simulink model "AEKF_Digital_Twin"  (R2026a)
settings: Solver=ode1  StopTime=T_sim  FixedStep=0.002
settings Model: Creator=Adham  LastModifiedBy=Adham

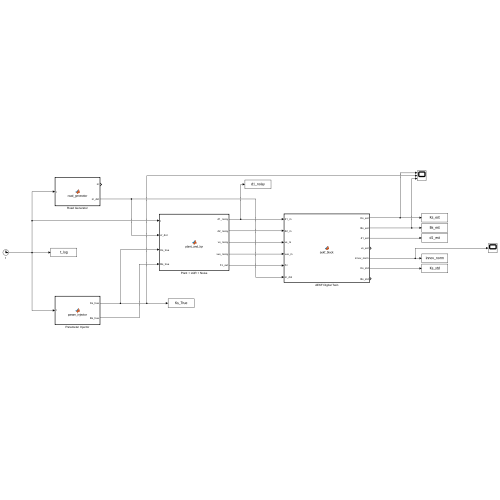
[thumbnail: Simulink's stored preview of the top-level diagram]
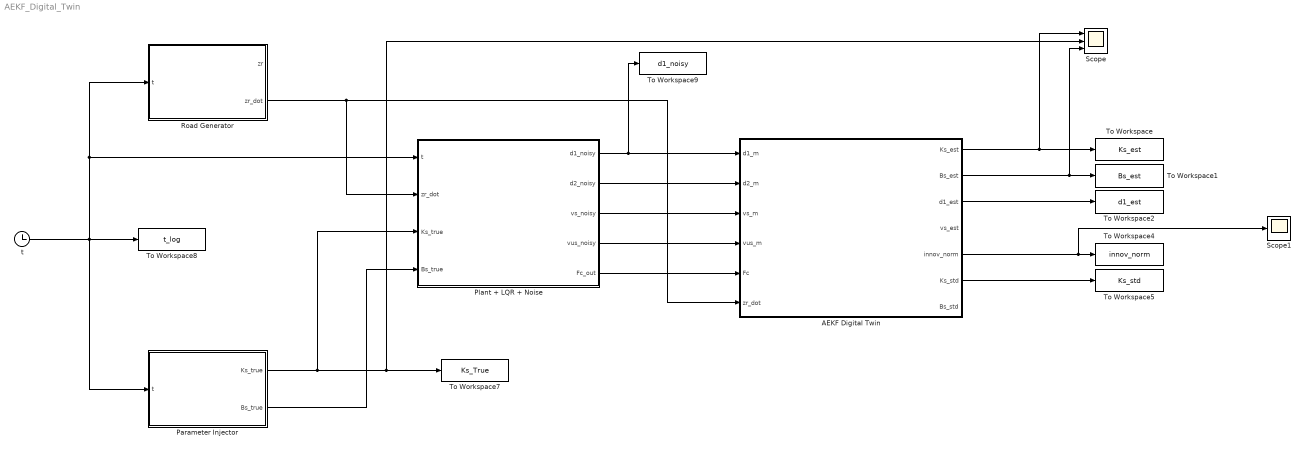
== system AEKF_Digital_Twin ==
  AEKF Digital Twin : MATLAB Function  TreatAsAtomicUnit=on
  Parameter Injector : MATLAB Function  TreatAsAtomicUnit=on
  Plant + LQR + Noise : MATLAB Function  TreatAsAtomicUnit=on
  Road Generator : MATLAB Function  TreatAsAtomicUnit=on
  Scope : Scope  NumInputPorts=3
  Scope1 : Scope
  To Workspace : ToWorkspace  VariableName=Ks_est  SaveFormat=Timeseries  SampleTime=-1
  To Workspace1 : ToWorkspace  VariableName=Bs_est  SaveFormat=Timeseries  SampleTime=-1
  To Workspace2 : ToWorkspace  VariableName=d1_est  SaveFormat=Timeseries  SampleTime=-1
  To Workspace4 : ToWorkspace  VariableName=innov_norm  SaveFormat=Timeseries  SampleTime=-1
  To Workspace5 : ToWorkspace  VariableName=Ks_std  SaveFormat=Timeseries  SampleTime=-1
  To Workspace7 : ToWorkspace  VariableName=Ks_True  SaveFormat=Timeseries  SampleTime=-1
  To Workspace8 : ToWorkspace  VariableName=t_log  SaveFormat=Timeseries  SampleTime=-1
  To Workspace9 : ToWorkspace  VariableName=d1_noisy  SaveFormat=Timeseries  SampleTime=-1
  t : Clock
  wires:
  t/1 -> To Workspace8/1, Road Generator/1(t), Plant + LQR + Noise/1(t), Parameter Injector/1(t)
  Parameter Injector/1(Ks_true) -> To Workspace7/1, Scope/2, Plant + LQR + Noise/3(Ks_true)
  Parameter Injector/2(Bs_true) -> Plant + LQR + Noise/4(Bs_true)
  Plant + LQR + Noise/1(d1_noisy) -> To Workspace9/1, AEKF Digital Twin/1(d1_m)
  Plant + LQR + Noise/2(d2_noisy) -> AEKF Digital Twin/2(d2_m)
  Plant + LQR + Noise/3(vs_noisy) -> AEKF Digital Twin/3(vs_m)
  Plant + LQR + Noise/4(vus_noisy) -> AEKF Digital Twin/4(vus_m)
  Plant + LQR + Noise/5(Fc_out) -> AEKF Digital Twin/5(Fc)
  Road Generator/2(zr_dot) -> AEKF Digital Twin/6(zr_dot), Plant + LQR + Noise/2(zr_dot)
  AEKF Digital Twin/1(Ks_est) -> Scope/1, To Workspace/1
  AEKF Digital Twin/2(Bs_est) -> Scope/3, To Workspace1/1
  AEKF Digital Twin/5(innov_norm) -> Scope1/1, To Workspace4/1
  AEKF Digital Twin/6(Ks_std) -> To Workspace5/1
  AEKF Digital Twin/3(d1_est) -> To Workspace2/1

== matlab function AEKF_Digital_Twin/Parameter Injector ==
  data: t input; Ks_true output; Bs_true output
function [Ks_true, Bs_true] = param_injector(t)
%#codegen
    Ks_1    = 900.0;   % N/m before change
    Ks_2    = 700.0;   % N/m after change
    t_chg   = 60.0;    % injection time
    Bs_true = 58.08;   % constant throughout
    
    if t < t_chg
        Ks_true = Ks_1;
    else
        Ks_true = Ks_2;
    end
end

== matlab function AEKF_Digital_Twin/Road Generator ==
  data: t input; zr output; zr_dot output
function [zr, zr_dot] = road_generator(t)
%#codegen
    RoadAmp  = 0.015;   % m
    RoadFreq = 25.0;    % rad/s
    zr     = RoadAmp * sin(RoadFreq * t);
    zr_dot = RoadAmp * RoadFreq * cos(RoadFreq * t);
end

== matlab function AEKF_Digital_Twin/Plant + LQR + Noise ==
  data: t input; d1_noisy output; zr_dot input; Ks_true input; Bs_true input; d2_noisy output; vs_noisy output; vus_noisy output; Fc_out output
function [d1_noisy, d2_noisy, vs_noisy, vus_noisy, Fc_out] = ...
    plant_and_lqr(t, zr_dot, Ks_true, Bs_true)
%#codegen

%% System parameters
Ms  = 2.45;    Mus = 1.00;
Kus = 1250.0;  Bus = 14.726;

%% LQR gain [reordered for state: d1, d2, vs, vus]
K_lqr = [11.3848, -206.1923, 61.4922, -4.4806];

%% Measurement noise std devs
sigma_d  = 0.001;   % 1 mm std for d1, d2
sigma_v  = 0.003;   % 3 mm/s std for vs, vus

dt = 0.002;

%% Persistent state (plant true state)
persistent x_plant;
if isempty(x_plant)
    x_plant = zeros(4,1);  % start at equilibrium
end

%% LQR control (uses true state — ideal scenario for validation)
Fc = -K_lqr * x_plant;
Fc = max(-50, min(50, Fc));   % saturate at ±50 N (realistic actuator limit)

%% RK4 plant integration
k1 = plant_f(x_plant, Fc, zr_dot, Ks_true, Bs_true, Ms, Mus, Kus, Bus);
k2 = plant_f(x_plant + 0.5*dt*k1, Fc, zr_dot, Ks_true, Bs_true, Ms, Mus, Kus, Bus);
k3 = plant_f(x_plant + 0.5*dt*k2, Fc, zr_dot, Ks_true, Bs_true, Ms, Mus, Kus, Bus);
k4 = plant_f(x_plant + dt*k3, Fc, zr_dot, Ks_true, Bs_true, Ms, Mus, Kus, Bus);
x_plant = x_plant + (dt/6)*(k1 + 2*k2 + 2*k3 + k4);

%% Add measurement noise
d1_noisy  = x_plant(1) + sigma_d * randn;
d2_noisy  = x_plant(2) + sigma_d * randn;
vs_noisy  = x_plant(3) + sigma_v * randn;
vus_noisy = x_plant(4) + sigma_v * randn;
Fc_out = Fc;

end

%% ===== LOCAL FUNCTION: Plant Dynamics =====
function dx = plant_f(x, Fc, zr_dot, Ks, Bs, Ms, Mus, Kus, Bus)
% State: [d1=zs-zus, d2=zus-zr, vs=żs, vus=żus]
dx = zeros(4,1);
dx(1) = x(3) - x(4);
dx(2) = x(4) - zr_dot;
dx(3) = -(Ks/Ms)*x(1) - (Bs/Ms)*(x(3)-x(4)) + Fc/Ms;
dx(4) = (Ks/Mus)*x(1) - (Kus/Mus)*x(2) + (Bs/Mus)*(x(3)-x(4)) ...
        - (Bus/Mus)*x(4) + (Bus/Mus)*zr_dot - Fc/Mus;
end

== matlab function AEKF_Digital_Twin/AEKF Digital Twin ==
  data: d1_m input; Ks_est output; d2_m input; vs_m input; vus_m input; Fc input; zr_dot input; Bs_est output; d1_est output; vs_est output; innov_norm output; Ks_std output; Bs_std output
function [Ks_est, Bs_est, d1_est, vs_est, innov_norm, Ks_std, Bs_std] = ...
    aekf_block(d1_m, d2_m, vs_m, vus_m, Fc, zr_dot)
%#codegen

%% System constants
Ms  = 2.45;    Mus = 1.00;
Kus = 1250.0;  Bus = 14.726;
dt  = 0.002;

%% Measurement noise R (fixed)
R_meas = diag([0.001^2, 0.001^2, 0.003^2, 0.003^2]);

%% Sage-Husa forgetting factor
b_sh = 0.97;

%% Persistent AEKF state
persistent x_aug P Q_adapt step_k;

if isempty(x_aug)
    x_aug  = [0; 0; 0; 0; 900.0; 58.08];  % [d1,d2,vs,vus,Ks,Bs]
    P      = diag([0.003^2, 0.003^2, 0.05^2, 0.05^2, 150^2, 20^2]);
    Q_adapt = diag([(2e-4)^2, (2e-4)^2, 0.01^2, 0.01^2, 5.0^2, 0.5^2]);
    step_k = int32(0);
end

%% ===== PREDICTION STEP =====
dx  = f_aug(x_aug, Fc, zr_dot, Ms, Mus, Kus, Bus);
x_aug = x_aug + dt * dx;

Fc_jac = F_jac(x_aug, Ms, Mus, Kus, Bus);
F_d = eye(6) + Fc_jac * dt;       % discrete Jacobian (Euler, valid at dt=0.002s)
P = F_d * P * F_d' + Q_adapt;
P = (P + P') * 0.5;               % enforce symmetry

%% ===== UPDATE STEP =====
H = [eye(4, 4), zeros(4, 2)];     % 4×6, linear measurement model

z = [d1_m; d2_m; vs_m; vus_m];   % measurement vector
innov = z - x_aug(1:4);           % 4×1 innovation

S = H * P * H' + R_meas;          % 4×4 innovation covariance
K = P * H' / S;                   % 6×4 Kalman gain

x_aug = x_aug + K * innov;        % state update

IKH = eye(6) - K * H;             % Joseph form (numerically stable)
P = IKH * P * IKH' + K * R_meas * K';
P = (P + P') * 0.5;

%% ===== SAGE-HUSA ADAPTIVE Q UPDATE =====
step_k = step_k + int32(1);
d_sh = (1.0 - b_sh) / (1.0 - b_sh^double(step_k));
Q_new = K * (innov * innov') * K';
Q_adapt = (1.0 - d_sh) * Q_adapt + d_sh * Q_new;

% Floor Q to prevent collapse
Q_floor = diag([1e-10, 1e-10, 1e-8, 1e-8, 0.1, 0.01]);
for i = 1:6
    if Q_adapt(i,i) < Q_floor(i,i)
        Q_adapt(i,i) = Q_floor(i,i);
    end
end

%% ===== PHYSICAL CONSTRAINTS ON PARAMETERS =====
if x_aug(5) < 50.0,  x_aug(5) = 50.0;   end  % Ks_min
if x_aug(6) < 0.5,   x_aug(6) = 0.5;    end  % Bs_min
if x_aug(5) > 2000.0, x_aug(5) = 2000.0; end  % Ks_max

%% ===== OUTPUTS =====
Ks_est    = x_aug(5);
Bs_est    = x_aug(6);
d1_est    = x_aug(1);
vs_est    = x_aug(3);
innov_norm = norm(innov);
Ks_std    = sqrt(P(5,5));
Bs_std    = sqrt(P(6,6));

end  % end main function

%% ===== LOCAL FUNCTION: Augmented Dynamics =====
function dx = f_aug(x, Fc, zr_dot, Ms, Mus, Kus, Bus)
Ks = x(5);   Bs = x(6);
dx = zeros(6,1);
dx(1) = x(3) - x(4);
dx(2) = x(4) - zr_dot;
dx(3) = -(Ks/Ms)*x(1) - (Bs/Ms)*(x(3)-x(4)) + Fc/Ms;
dx(4) = (Ks/Mus)*x(1) - (Kus/Mus)*x(2) + (Bs/Mus)*(x(3)-x(4)) ...
        - (Bus/Mus)*x(4) + (Bus/Mus)*zr_dot - Fc/Mus;
dx(5) = 0;   % Ks: random walk
dx(6) = 0;   % Bs: random walk
end

%% ===== LOCAL FUNCTION: Jacobian of Augmented Dynamics =====
function F = F_jac(x, Ms, Mus, Kus, Bus)
Ks = x(5);   Bs = x(6);
F = zeros(6,6);
%--- Row 1: ∂(ẋ1)/∂x ---
F(1,3) =  1;     F(1,4) = -1;
%--- Row 2: ∂(ẋ2)/∂x ---
F(2,4) =  1;
%--- Row 3: ∂(ẋ3)/∂x ---
F(3,1) = -Ks/Ms;   F(3,3) = -Bs/Ms;   F(3,4) =  Bs/Ms;
F(3,5) = -x(1)/Ms; F(3,6) = -(x(3)-x(4))/Ms;
%--- Row 4: ∂(ẋ4)/∂x ---
F(4,1) =  Ks/Mus;  F(4,2) = -Kus/Mus;
F(4,3) =  Bs/Mus;  F(4,4) = -(Bs+Bus)/Mus;
F(4,5) =  x(1)/Mus; F(4,6) = (x(3)-x(4))/Mus;
%--- Rows 5,6: parameters are random walks, Jacobian = 0 ---
end
